simulink model "FirstOrderModelDelayed"  (R2021b)
settings: Solver=VariableStepAuto  StartTime=0.0  StopTime=50  RelTol=1e-3
undefined symbols (not defined in the file): delay, k, tau
settings Model: Creator=Jonah  LastModifiedBy=Jonah

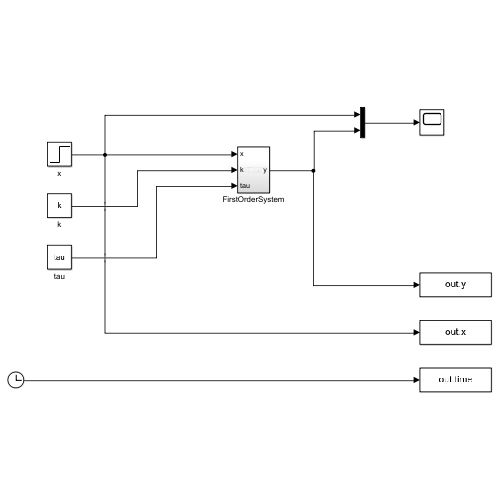
[thumbnail: Simulink's stored preview of the top-level diagram]
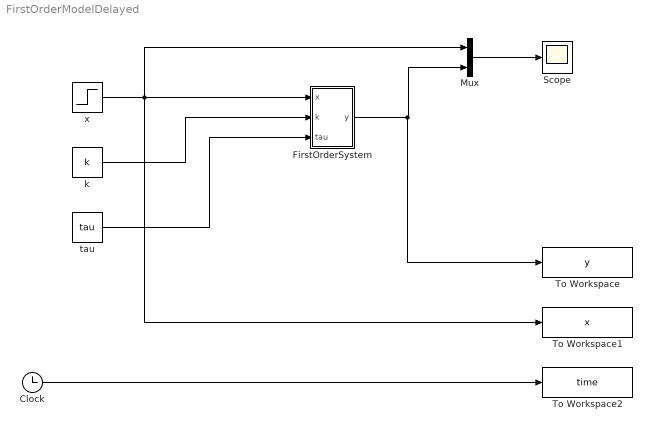
== system FirstOrderModelDelayed ==
  Clock : Clock
  FirstOrderSystem : Subsystem
  Mux : Mux  Inputs=2
  Scope : Scope
  To Workspace : ToWorkspace  VariableName=y  SampleTime=-1
  To Workspace1 : ToWorkspace  VariableName=x  SampleTime=-1
  To Workspace2 : ToWorkspace  VariableName=time  SampleTime=-1
  k : Constant  Value=k
  tau : Constant  Value=tau
  x : Step  Time=delay  SampleTime=0
  wires:
  x/1 -> To Workspace1/1, Mux/1, FirstOrderSystem/1(x)
  k/1 -> FirstOrderSystem/2(k)
  Mux/1 -> Scope/1
  FirstOrderSystem/1(y) -> To Workspace/1, Mux/2
  Clock/1 -> To Workspace2/1
  tau/1 -> FirstOrderSystem/3(tau)

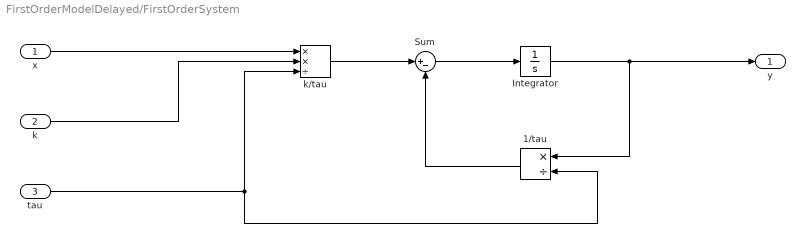
== system FirstOrderModelDelayed/FirstOrderSystem ==
  x : Inport
  k : Inport  Port=2
  tau : Inport  Port=3
  1/tau : Product  Inputs=*/
  Integrator : Integrator
  Sum : Sum  Inputs=|+-
  k/tau : Product  Inputs=**/
  y : Outport
  wires:
  Integrator/1 -> y/1, 1/tau/1
  tau/1 -> k/tau/3, 1/tau/2
  Sum/1 -> Integrator/1
  1/tau/1 -> Sum/2
  k/1 -> k/tau/2
  k/tau/1 -> Sum/1
  x/1 -> k/tau/1
